simulink model "ad9361_tx_model"  (R2017b)
settings: Solver=ode23tb  StartTime=0.0  StopTime=inf  RelTol=1e-3  EnableMultiTasking=on
PreLoadFcn:
  | ad9361_preload(bdroot,'tx')
undefined symbols (not defined in the file or in its folder): magnitude, var
libraries: dspsrcs4 x5, dspmathops x3, ad9361_models x1
CloseFcn:
  | clear ad9361_tx_hm1Filt ad9361_tx_hm2Filt;
  | clear ad9361_tx_hm3Filt ad9361_tx_hm4Filt;
settings Model: SimulationMode=accelerator  NumberOfSteps=100  Creator=The MathWorks Inc.  LastModifiedBy=ppradhan
settings DataIOCC: ExternalInput=txWaveform  SaveFormat=StructureWithTime  SaveOutput=off  SignalLogging=off  DSMLogging=off  SaveTime=off  OutputSaveName=rx
settings OptimizationCC: DefaultParameterBehavior=Inlined  InlineInvariantSignals=on  EfficientMapNaN2IntZero=off  LifeSpan=inf  SimCompilerOptimization=on
settings DebuggingCC: UnderspecifiedInitializationDetection=Classic  MergeDetectMultiDrivingBlocksExec=none  SolverPrmCheckMsg=warning  MultiTaskDSMMsg=warning  MultiTaskCondExecSysMsg=none  AllowSymbolicDim=off  SFUnexpectedBacktrackingDiag=warning  SFNoUnconditionalDefaultTransitionDiag=none  SFUndirectedBroadcastEventsDiag=none  SFExecutionAtInitializationDiag=none
settings HardwareCC: ProdBitPerPointer=32  ProdBitPerSizeT=32  ProdBitPerPtrDiffT=32  ProdLargestAtomicFloat=None  ProdIntDivRoundTo=Undefined  ProdEndianess=Unspecified  ProdWordSize=32  ProdHWDeviceType=32-bit Generic  TargetBitPerPointer=64  TargetBitPerSizeT=64  TargetBitPerPtrDiffT=64  TargetLongLongMode=on  TargetIntDivRoundTo=Zero  TargetEndianess=LittleEndian  TargetWordSize=64  TargetHWDeviceType=MATLAB Host  ProdEqTarget=off
settings ModelReferenceCC: PropagateSignalLabelsOutOfModel=off
settings CodeAppCC: MaxIdLength=128  StateflowObjectComments=on
settings GRTTargetCC: TargetLangStandard=C89/C90 (ANSI)  CombineOutputUpdateFcns=off  GRTInterface=on
settings ConfigComp: CovMetricSettings=dw  CovHtmlReporting=on  CovSaveCumulativeToWorkspaceVar=on  CovSaveSingleToWorkspaceVar=on  CovShowResultsExplorer=off  CovExternalEMLEnable=off  CovSFcnEnable=off
settings SimscapeCC: ExplicitSolverDiagnosticOptions=none

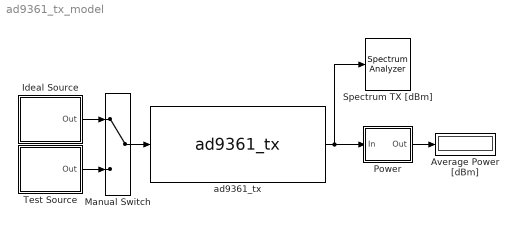
== system ad9361_tx_model ==
  Average Power [dBm] : Display
  Ideal Source : Subsystem  mask{Sel=Single CW tone, CW=2e6, Pow=0, Tstep=1.302083333333333e-07}
      mask prompts: Sel "Select Source"; CW "Frequency (Hz)"; Pow "Power (dBFS)"; Tstep "Sample Time (s)"
      mask TypeOptions Sel: CW + 1MHz tone | Single CW tone | Dual CW tone
      mask DialogControl DescGroupVar Prompt: Ideal Test Source
      mask Display: disp('CW Source')
  Manual Switch : ManualSwitch
  Power : Subsystem  mask{R=1}
      mask prompts: R "Reference Impedance [Ohm]"
      mask DialogControl DescGroupVar Prompt: Power Meter
      mask Display: disp('Power \nMeter');
  Spectrum TX [dBm] : SpectrumAnalyzer
  Test Source : Subsystem  mask{TestSignal=5MHz LTE-like test signal, TxCustVector=complex(rand(1000,1), rand(1000,1)), Tstep=1.302083333333333e-07, LTE_Pow=0}
      mask prompts: TestSignal "Test Signal"; TxCustVector "Custom Test Vector Complex data (I, Q)"; Tstep "Sample Time (sec)"; LTE_Pow "Relative Power scaling (dBFS)"
      mask init:
      | %disp(['Start initialization ' get_param(gcb,'TestSignal')])
      | load ad9361_LTE_data;
      | if strcmpi(TestSignal,'5MHz LTE-like test signal')
      |     tx = tx5;
      |     LTE = 5;
      |     SampleTime = 1/info5.SamplingRate;
      |     set_param(gcb,'Tstep',num2str(SampleTime,16));
      | elseif strcmpi(TestSignal,'10MHz LTE-like test signal')
      |     tx = tx10;
      |     LTE = 10;
      |     SampleTime = 1/info10.SamplingRate;
      |     set_param(gcb,'Tstep',num2str(SampleTime,16));
      | elseif strcmpi(TestSignal,'20MHz LTE-like test signal')
      |     tx = tx20;
      |     LTE = 20;
      |     SampleTime = 1/info20.SamplingRate;
      |     set_param(gcb,'Tstep',num2str(SampleTime,16));
      | elseif strcmpi(TestSignal,'Custom Signal')
      |     LTE = 0;
      |     tx = TxCustVector;
      |     SampleTime = str2num(get_param(gcb,'Tstep'));
      | else
      |     error(message('rfblks_adiagile:adiagile:UnknownTestSig',gcb,TestSignal));
      | end
      | idlSrc = [bdroot '/Ideal Source'];
      | set_param(idlSrc,'Tstep',num2str(SampleTime,16));
      | 
      | p = Simulink.Mask.get(gcb);
      | p.Parameters(3).Value = num2str(SampleTime,16);
      | %disp(['End initialization ' num2str(get_param(gcb,'Tstep'))])
      mask TypeOptions TestSignal: 5MHz LTE-like test signal | 10MHz LTE-like test signal | 20MHz LTE-like test signal | Custom signal
      mask Callback TestSignal:
      | % Set Mask visibilites and enables
      | ad9361_tx_mask_callbacks(gcb,'TestSigType')
      mask DialogControl DescGroupVar Prompt: Test Source TX
      mask Display: disp('LTE Source')
  ad9361_tx : ad9361_models/ad9361_tx  TestSignal=5MHz LTE  LOFreq=2e9
      settings: SourceProductName=RF Blockset Models for Analog Devices RF Transceivers
  wires:
  Test Source/1(Out) -> Manual Switch/2
  Ideal Source/1(Out) -> Manual Switch/1
  Power/1(Out) -> Average Power [dBm]/1
  ad9361_tx/1 -> Power/1(In), Spectrum TX [dBm]/1
  Manual Switch/1 -> ad9361_tx/1

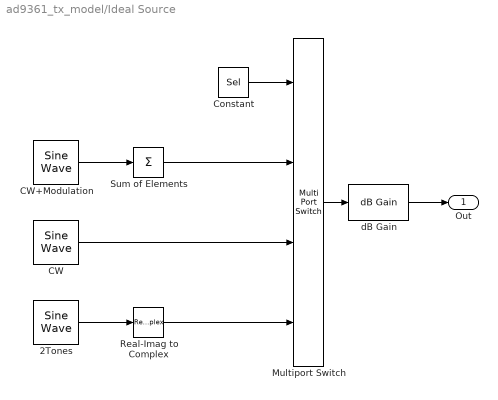
== system ad9361_tx_model/Ideal Source ==
  2Tones : dspsrcs4/Sine Wave  Amplitude=sqrt(2)  Frequency=CW/2  Phase=0  SampleMode=Discrete  OutComplex=Real  CompMethod=Trigonometric fcn  TableSize=Speed  SampleTime=Tstep  SamplesPerFrame=1  ResetState=Restart at time zero  OutputFrames=on  dataType=double  wordLen=16  udDataType=sfix(16)  fracBitsMode=Best precision  numFracBits=15  OutDataTypeStr=double  LastOutDataTypeStr=double
  CW : dspsrcs4/Sine Wave  Amplitude=1  Frequency=CW  Phase=0  SampleMode=Discrete  OutComplex=Complex  CompMethod=Trigonometric fcn  TableSize=Speed  SampleTime=Tstep  SamplesPerFrame=1  ResetState=Restart at time zero  OutputFrames=on  dataType=double  wordLen=16  udDataType=sfix(16)  fracBitsMode=Best precision  numFracBits=15  OutDataTypeStr=double  LastOutDataTypeStr=double
  CW+Modulation : dspsrcs4/Sine Wave  Amplitude=[1; 1]/sqrt(2)  Frequency=[CW; 1e6]  Phase=[0; 0]  SampleMode=Discrete  OutComplex=Complex  CompMethod=Trigonometric fcn  TableSize=Speed  SampleTime=Tstep  SamplesPerFrame=1  ResetState=Restart at time zero  OutputFrames=on  dataType=double  wordLen=16  udDataType=sfix(16)  fracBitsMode=Best precision  numFracBits=15  OutDataTypeStr=double  LastOutDataTypeStr=double
  Constant : Constant  Value=Sel  SampleTime=Tstep
  Multiport Switch : MultiPortSwitch
  Real-Imag to Complex : RealImagToComplex  Input=Real
  Sum of Elements : Sum  Inputs=+
  dB Gain : dspmathops/dB Gain  dB=Pow-30  intype=Amplitude
      settings: SourceProductName=DSP System Toolbox  SourceProductBaseCode=DS
  Out : Outport
  wires:
  CW+Modulation/1 -> Sum of Elements/1
  Sum of Elements/1 -> Multiport Switch/2
  CW/1 -> Multiport Switch/3
  2Tones/1 -> Real-Imag to Complex/1
  Constant/1 -> Multiport Switch/1
  Real-Imag to Complex/1 -> Multiport Switch/4
  Multiport Switch/1 -> dB Gain/1
  dB Gain/1 -> Out/1

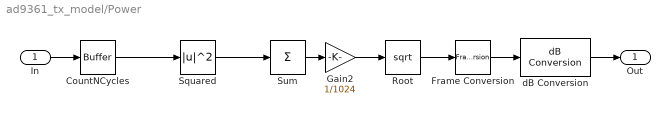
== system ad9361_tx_model/Power ==
  In : Inport
  CountNCycles : Buffer  N=1024
  Frame Conversion : FrameConversion  InheritSamplingMode=off  OutFrame=Sample-based
  Gain2 : Gain  Gain=1/1024
  Root : Sqrt  SaturateOnIntegerOverflow=on
  Squared : Math  Operator=magnitude^2  SaturateOnIntegerOverflow=on
  Sum : Sum  Inputs=+
  dB Conversion : dspmathops/dB Conversion  dBtype=dBm  intype=Amplitude  R=R  fuzz=on
      settings: SourceProductName=DSP System Toolbox
  Out : Outport
  wires:
  dB Conversion/1 -> Out/1
  In/1 -> CountNCycles/1
  Frame Conversion/1 -> dB Conversion/1
  CountNCycles/1 -> Squared/1
  Squared/1 -> Sum/1
  Sum/1 -> Gain2/1
  Root/1 -> Frame Conversion/1
  Gain2/1 -> Root/1

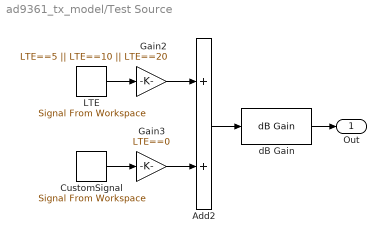
== system ad9361_tx_model/Test Source ==
  Add2 : Sum
  CustomSignal : dspsrcs4/Signal From Workspace  X=tx  Ts=Tstep  nsamps=1  OutputAfterFinalValue=Cyclic repetition  ignoreOrWarnInputAndFrameLengths=off  OutputFrames=on
  Gain2 : Gain  Gain=LTE==5 || LTE==10 || LTE==20
  Gain3 : Gain  Gain=LTE==0
  LTE : dspsrcs4/Signal From Workspace  X=tx  Ts=Tstep  nsamps=1  OutputAfterFinalValue=Cyclic repetition  ignoreOrWarnInputAndFrameLengths=off  OutputFrames=on
  dB Gain : dspmathops/dB Gain  dB=LTE_Pow-7-(10*log10(var(tx))+30)  intype=Amplitude
      settings: SourceProductName=DSP System Toolbox  SourceProductBaseCode=DS
  Out : Outport
  wires:
  LTE/1 -> Gain2/1
  Gain2/1 -> Add2/1
  CustomSignal/1 -> Gain3/1
  Add2/1 -> dB Gain/1
  Gain3/1 -> Add2/2
  dB Gain/1 -> Out/1
